simulink model "ISA_simulation"  (R2018b)
settings: Solver=FixedStepDiscrete  StartTime=0.0  StopTime=10  FixedStep=0.01  RelTol=1e-3
PreLoadFcn:
  | librarySetup
  | eval([bdroot,'_startup']) %Calling [modelName]_startup.m
InitFcn:
  | ISA_simulation_startup
values from neighbouring files (symbols this model uses):
  Error_detection = -1    [ISA_simulation_startup.m]
  ID727_Byte0 = 50    [ISA_simulation_startup.m]
  ID727_Byte1 = 0    [ISA_simulation_startup.m]
  ID727_Byte2 = 0    [ISA_simulation_startup.m]
  ID727_Byte3 = 0    [ISA_simulation_startup.m]
  ID727_Byte4 = 0    [ISA_simulation_startup.m]
  ID727_Byte5 = 0    [ISA_simulation_startup.m]
  ID727_Byte6 = 0    [ISA_simulation_startup.m]
  ID727_Byte7 = 0    [ISA_simulation_startup.m]
  ID7E8_Byte0 = 3    [ISA_simulation_startup.m]
  ID7E8_Byte1 = 65    [ISA_simulation_startup.m]
  ID7E8_Byte2 = 13    [ISA_simulation_startup.m]
  ID7E8_Byte3 = 2    [ISA_simulation_startup.m]
  ID7E8_Byte4 = 0    [ISA_simulation_startup.m]
  ID7E8_Byte5 = 0    [ISA_simulation_startup.m]
  ID7E8_Byte6 = 0    [ISA_simulation_startup.m]
  ID7E8_Byte7 = 0    [ISA_simulation_startup.m]
  PWM_motor = 0.6    [ISA_simulation_startup.m]    (also in ISA_startup.m = 0.55)
undefined symbols (not defined in the file or in its folder): DiscIntNeverNeededParam
libraries: simulink x14, HANcoder_STM32_Target x5, HANcoder_STM32_Target2009b x2, simulink_extras x1
CloseFcn:
  | rtwprivate ssgencode ModelCloseRequest mytest
settings Model: Creator=Saliou  LastModifiedBy=Saliou
settings SolverCC: PositivePriorityOrder=on
settings DataIOCC: LimitDataPoints=on  SaveFormat=Array  SaveOutput=off  SaveTime=off
settings OptimizationCC: BlockReduction=off  DefaultParameterBehavior=Inlined  DefaultUnderspecifiedDataType=single  InlineInvariantSignals=on  ExpressionDepthLimit=2147483647  StateBitsets=on  DataBitsets=on  ZeroExternalMemoryAtStartup=off  ZeroInternalMemoryAtStartup=off  InitFltsAndDblsToZero=on  NoFixptDivByZeroProtection=on  EfficientFloat2IntCast=on  LifeSpan=inf
settings DebuggingCC: SaveWithDisabledLinksMsg=none  SaveWithParameterizedLinksMsg=none  CheckSSInitialOutputMsg=off  UnderspecifiedInitializationDetection=Classic  MergeDetectMultiDrivingBlocksExec=none  SignalResolutionControl=TryResolveAll  SolverPrmCheckMsg=warning  InheritedTsInSrcMsg=none  MultiTaskDSMMsg=warning  MultiTaskCondExecSysMsg=none  ParameterPrecisionLossMsg=none  FcnCallInpInsideContextMsg=warning  StateNameClashWarn=warning  SFUnexpectedBacktrackingDiag=warning  SFNoUnconditionalDefaultTransitionDiag=warning  SFExecutionAtInitializationDiag=none
settings HardwareCC: ProdBitPerPointer=32  ProdBitPerSizeT=32  ProdBitPerPtrDiffT=32  ProdLargestAtomicInteger=Long  ProdLargestAtomicFloat=Double  ProdWordSize=32  ProdHWDeviceType=ARM Compatible->ARM Cortex  TargetEndianess=LittleEndian  TargetHWDeviceType=Infineon->TriCore
settings ModelReferenceCC: PropagateSignalLabelsOutOfModel=off
settings SFSimCC: SimUseLocalCustomCode=off  MATLABDynamicMemAlloc=off
settings RTWCC: SystemTargetFile=ert.tlc  MakeCommand=make_rtw SHELL= HANcoder_PORTABLE=1 HANcoder_BOOTLOADER=1  TemplateMakefile=Olimexino_STM32_gcc.tmf  Description=Real-Time Workshop Embedded Coder (no auto configuration)  RTWUseLocalCustomCode=off
settings CodeAppCC: ForceParamTrailComments=on  IgnoreCustomStorageClasses=off  SimulinkDataObjDesc=on  CustomSymbolStrGlobalVar=rt$N$M  CustomSymbolStrType=$N$M  CustomSymbolStrFcn=$N$M$F  CustomSymbolStrMacro=$N$M  InsertBlockDesc=on  StateflowObjectComments=on  InternalIdentifier=Classic
settings ERTTargetCC: TargetFcnLib=ansi_tfl_tmw.mat  MultiwordLength=2048  IncludeMdlTerminateFcn=off  SuppressErrorStatus=on  SupportNonFinite=off  GenerateASAP2=on  InlinedParameterPlacement=NonHierarchical  ERTCustomFileTemplate=example_file_process.tlc  ConvertIfToSwitch=off  SuppressUnreachableDefaultCases=off
settings ConfigComp: CovMetricSettings=dw  CovHtmlReporting=on  CovSaveCumulativeToWorkspaceVar=on  CovSaveSingleToWorkspaceVar=on  CovExternalEMLEnable=off  CovSFcnEnable=off  DVMaxProcessTime=600  DVDisplayUnsatisfiableObjectives=on  DVAutomaticStubbing=off  DVModelCoverageObjectives=MCDC  DVMaxTestCaseSteps=500  DVTestSuiteOptimization=CombinedObjectives  DVDetectActiveLogic=on  DVSaveHarnessModel=on

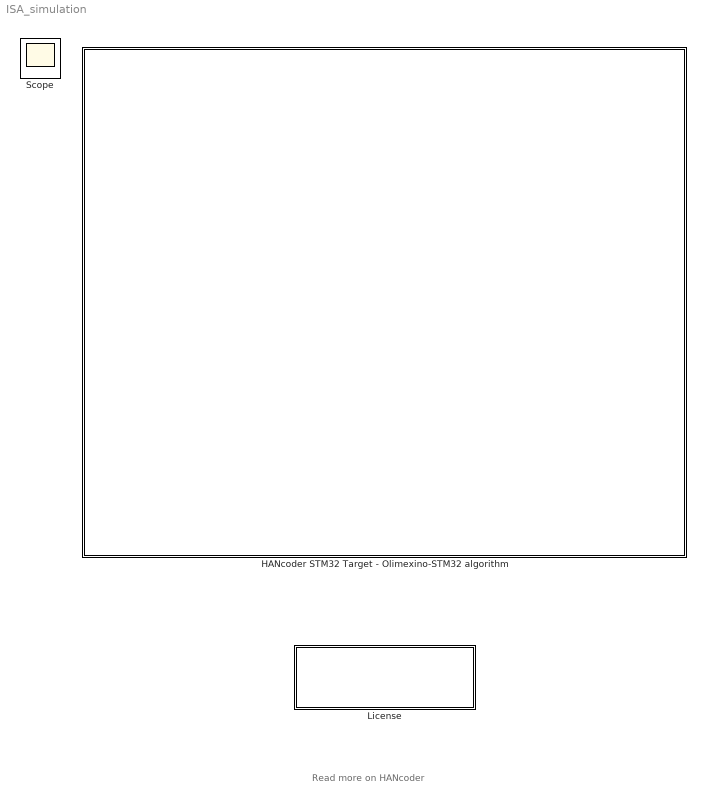
== system ISA_simulation ==
  note: Read more on HANcoder
  HANcoder STM32 Target - Olimexino-STM32 algorithm : Subsystem  mask(TopLevelSubsystem){}
      settings: CopyFcn=HANcoderChecks('Copy');  NameChangeFcn=HANcoderChecks('NameChangeOlimexino');  MoveFcn=HANcoderChecks('MoveOlimexino');
      mask Display: image(imread('Olimexino_STM32_HAN.jpg'))
  License : Subsystem  mask(License){}
      settings: NameChangeFcn=HANcoderChecks('NameChangeLicenseBlock');  OpenFcn=winopen('License.pdf')  MoveFcn=HANcoderChecks('MoveLicenseBlock');
      mask Display: disp(['End-User License Agreement\n','please read before use']);
  Scope : Scope

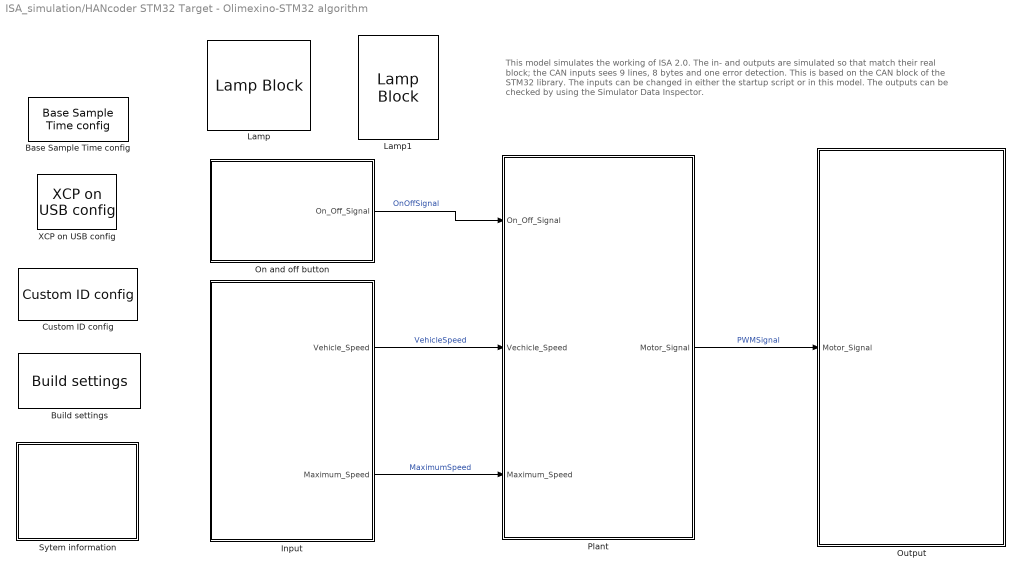
== system ISA_simulation/HANcoder STM32 Target - Olimexino-STM32 algorithm ==
  note: This model simulates the working of ISA 2.0. The in- and outputs are simulated so that match their real
      | block; the CAN inputs sees 9 lines, 8 bytes and one error detection. This is based on the CAN block of the
      | STM32 library. The inputs can be changed in either the startup script or in this model. The outputs can be
      | checked by using the Simulator Data Inspector.
  Base Sample Time config : HANcoder_STM32_Target/Olimexino STM32/System Config/Base Sample Time config  Tag=HANcoder_TARGET_STM32_Olimexino  Description=HANcoder Target STM32-Olimexino blockset version 1.0  baseSampleTime=10  extraStack=0
      settings: SourceProductName=HANcoder STM32 Target
  Build settings : HANcoder_STM32_Target/Olimexino STM32/System Config/Build settings  Tag=HANcoder_TARGET_STM32_Olimexino  AutoASAP2add=on  AutoFlash=USB
      settings: SourceProductName=HANcoder STM32 Target
  Custom ID config : HANcoder_STM32_Target2009b/Olimexino STM32/System Config/Custom ID config  Tag=HANcoder_TARGET_STM32_Olimexino  softID=softwareID  softNUM=1
  Input : Subsystem
  Lamp : LampBlock  WebBlockId=3805
  Lamp1 : LampBlock  WebBlockId=3832
  On and off button : Subsystem
  Output : Subsystem
  Plant : Subsystem
  Sytem information : Subsystem
  XCP on USB config : HANcoder_STM32_Target2009b/Olimexino STM32/System Config/XCP on USB config  Tag=HANcoder_TARGET_STM32_Olimexino
  wires:
  Input/2(Maximum_Speed) -> Plant/3(Maximum_Speed)  "MaximumSpeed"
  Input/1(Vehicle_Speed) -> Plant/2(Vechicle_Speed)  "VehicleSpeed"
  Plant/1(Motor_Signal) -> Output/1(Motor_Signal)  "PWMSignal"
  On and off button/1(On_Off_Signal) -> Plant/1(On_Off_Signal)  "OnOffSignal"

== system ISA_simulation/License ==

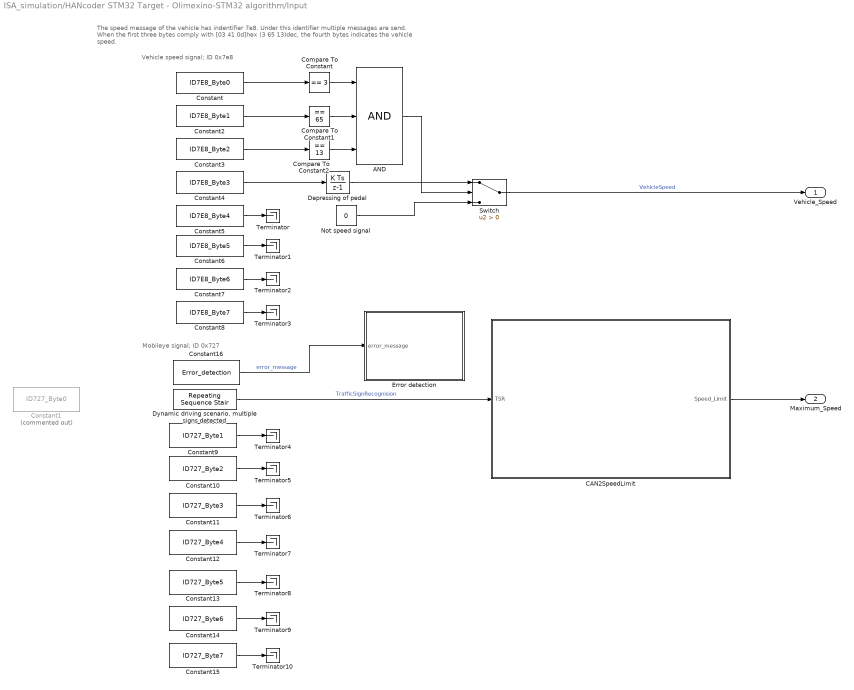
== system ISA_simulation/HANcoder STM32 Target - Olimexino-STM32 algorithm/Input ==
  note: Mobileye signal; ID 0x727
  note: Vehicle speed signal; ID 0x7e8
  note: The speed message of the vehicle has indentifier 7e8. Under this identifier multiple messages are send. When the first three bytes comply with [03 41 0d]hex (3 65 13)dec, the fourth bytes indicates the vehicle speed.
  AND : Logic  Inputs=3  AllPortsSameDT=off  OutDataTypeStr=boolean
  CAN2SpeedLimit : Subsystem
  Compare To Constant : simulink/Logic and Bit Operations/Compare To Constant  relop===  const=3  OutDataTypeStr=boolean
  Compare To Constant1 : simulink/Logic and Bit Operations/Compare To Constant  relop===  const=65  OutDataTypeStr=boolean
  Compare To Constant2 : simulink/Logic and Bit Operations/Compare To Constant  relop===  const=13  OutDataTypeStr=boolean
  Constant : Constant  Value=ID7E8_Byte0
  Constant1 : Constant  Commented=on  Value=ID727_Byte0  OutDataTypeStr=single
  Constant10 : Constant  Value=ID727_Byte2  OutDataTypeStr=single
  Constant11 : Constant  Value=ID727_Byte3  OutDataTypeStr=single
  Constant12 : Constant  Value=ID727_Byte4  OutDataTypeStr=single
  Constant13 : Constant  Value=ID727_Byte5  OutDataTypeStr=single
  Constant14 : Constant  Value=ID727_Byte6  OutDataTypeStr=single
  Constant15 : Constant  Value=ID727_Byte7  OutDataTypeStr=single
  Constant16 : Constant  Value=Error_detection  OutDataTypeStr=single
  Constant2 : Constant  Value=ID7E8_Byte1
  Constant3 : Constant  Value=ID7E8_Byte2
  Constant4 : Constant  Value=ID7E8_Byte3  OutDataTypeStr=single
  Constant5 : Constant  Value=ID7E8_Byte4  OutDataTypeStr=single
  Constant6 : Constant  Value=ID7E8_Byte5  OutDataTypeStr=single
  Constant7 : Constant  Value=ID7E8_Byte6  OutDataTypeStr=single
  Constant8 : Constant  Value=ID7E8_Byte7  OutDataTypeStr=single
  Constant9 : Constant  Value=ID727_Byte1  OutDataTypeStr=single
  Depressing of pedal : DiscreteIntegrator  gainval=13  SampleTime=-1  ICPrevOutput=DiscIntNeverNeededParam  ICPrevScaledInput=DiscIntNeverNeededParam
  "Dynamic driving scenario, multiple signs detected" : simulink/Sources/Repeating Sequence Stair  OutValues=[2 7 4 12 9].'  tsamp=1  OutMin=[]  OutMax=[]  OutDataTypeStr=double  OutputDataTypeScalingMode=double  OutDataType=fixdt(0,8)  ConRadixGroup=Best Precision: Vector-wise  OutScaling=2^-12
  Error detection : Subsystem
  Not speed signal : Constant  Value=0
  Switch : Switch  Criteria=u2 > Threshold
  Terminator{,1..10} (11 alike) : Terminator
  Vehicle_Speed : Outport
  Maximum_Speed : Outport  Port=2
  wires:
  Switch/1 -> Vehicle_Speed/1  "VehicleSpeed"
  Constant/1 -> Compare To Constant/1
  Constant2/1 -> Compare To Constant1/1
  Constant3/1 -> Compare To Constant2/1
  Compare To Constant2/1 -> AND/3
  Compare To Constant1/1 -> AND/2
  Compare To Constant/1 -> AND/1
  AND/1 -> Switch/2
  Not speed signal/1 -> Switch/3
  Constant5/1 -> Terminator/1
  Constant6/1 -> Terminator1/1
  Constant7/1 -> Terminator2/1
  Constant8/1 -> Terminator3/1
  Constant9/1 -> Terminator4/1
  Constant10/1 -> Terminator5/1
  Constant11/1 -> Terminator6/1
  Constant12/1 -> Terminator7/1
  Constant13/1 -> Terminator8/1
  Constant14/1 -> Terminator9/1
  Constant15/1 -> Terminator10/1
  Constant4/1 -> Depressing of pedal/1
  Depressing of pedal/1 -> Switch/1
  "Dynamic driving scenario, multiple signs detected"/1 -> CAN2SpeedLimit/1(TSR)  "TrafficSignRecognision"
  CAN2SpeedLimit/1(Speed_Limit) -> Maximum_Speed/1
  Constant16/1 -> Error detection/1(error_message)  "error_message"

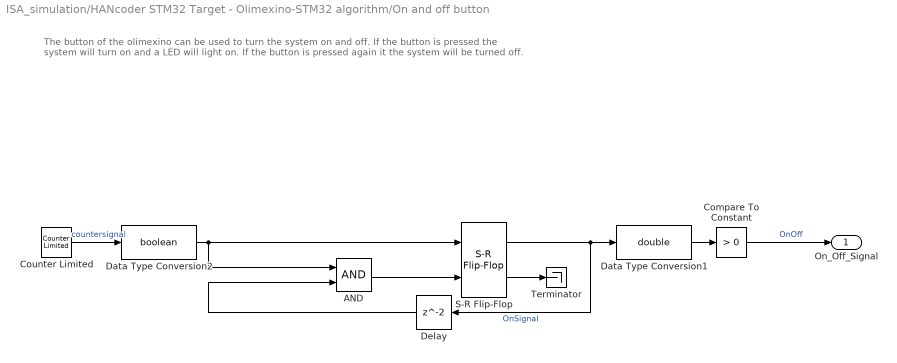
== system ISA_simulation/HANcoder STM32 Target - Olimexino-STM32 algorithm/On and off button ==
  note: The button of the olimexino can be used to turn the system on and off. If the button is pressed the system will turn on and a LED will light on. If the button is pressed again it the system will be turned off.
  AND : Logic  AllPortsSameDT=off  OutDataTypeStr=boolean
  Compare To Constant : simulink/Logic and Bit Operations/Compare To Constant  relop=>  const=0  OutDataTypeStr=boolean
  Counter Limited : simulink/Sources/Counter Limited  uplimit=1  tsamp=1
  Data Type Conversion1 : DataTypeConversion  OutDataTypeStr=double
  Data Type Conversion2 : DataTypeConversion  OutDataTypeStr=boolean
  Delay : Delay
  S-R Flip-Flop : simulink_extras/Flip Flops/S-R Flip-Flop  initial_condition=0
  Terminator : Terminator
  On_Off_Signal : Outport
  wires:
  AND/1 -> S-R Flip-Flop/2
  Data Type Conversion2/1 -> AND/1, S-R Flip-Flop/1
  Counter Limited/1 -> Data Type Conversion2/1  "countersignal"
  S-R Flip-Flop/1 -> Delay/1, Data Type Conversion1/1  "OnSignal"
  Data Type Conversion1/1 -> Compare To Constant/1
  Compare To Constant/1 -> On_Off_Signal/1  "OnOff"
  S-R Flip-Flop/2 -> Terminator/1
  Delay/1 -> AND/2

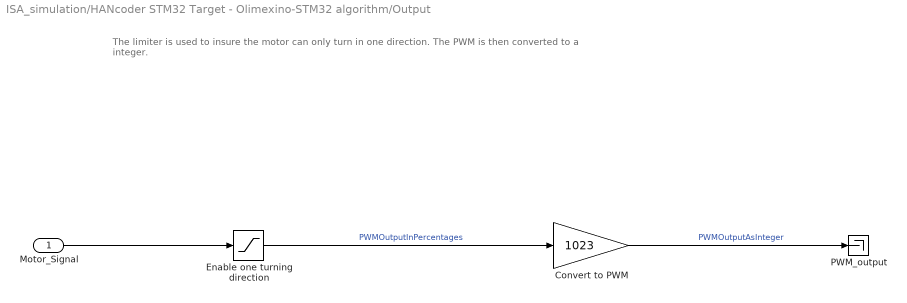
== system ISA_simulation/HANcoder STM32 Target - Olimexino-STM32 algorithm/Output ==
  note: The limiter is used to insure the motor can only turn in one direction. The PWM is then converted to a integer.
  Motor_Signal : Inport
  Convert to PWM : Gain  Gain=1023
  Enable one turning direction : Saturate  UpperLimit=0.6  LowerLimit=0
  PWM_output : Terminator
  wires:
  Motor_Signal/1 -> Enable one turning direction/1
  Enable one turning direction/1 -> Convert to PWM/1  "PWMOutputInPercentages"
  Convert to PWM/1 -> PWM_output/1  "PWMOutputAsInteger"

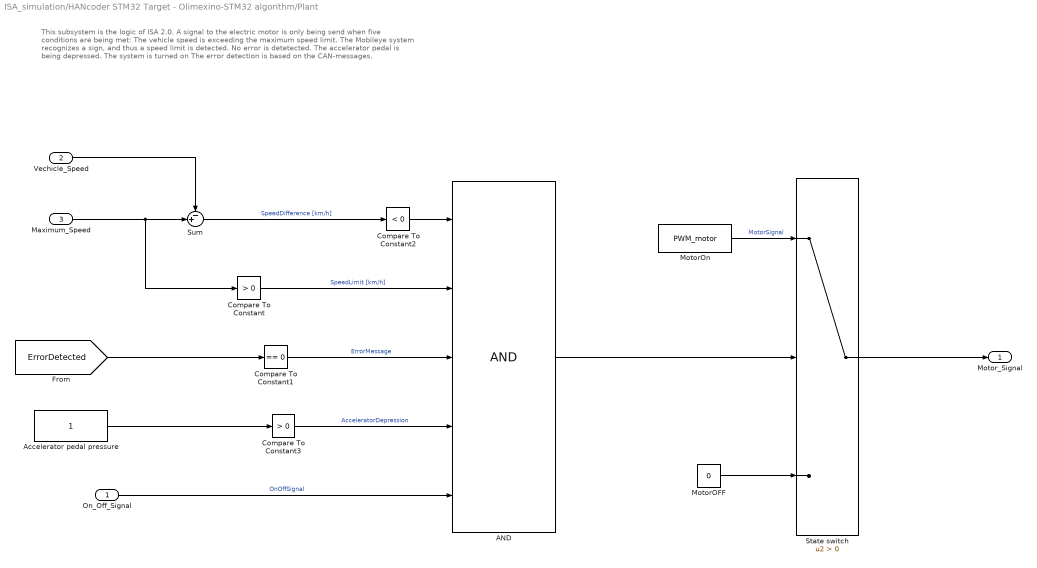
== system ISA_simulation/HANcoder STM32 Target - Olimexino-STM32 algorithm/Plant ==
  note: This subsystem is the logic of ISA 2.0. A signal to the electric motor is only being send when five conditions are being met:
      | The vehicle speed is exceeding the maximum speed limit.
      | The Mobileye system recognizes a sign, and thus a speed limit is detected.
      | No error is detetected.
      | The accelerator pedal is being depressed.
      | The system is turned on
      | The error detection is based on the CAN-messages.
  On_Off_Signal : Inport
  Vechicle_Speed : Inport  Port=2
  Maximum_Speed : Inport  Port=3
  AND : Logic  Inputs=5  AllPortsSameDT=off  OutDataTypeStr=boolean
  Accelerator pedal pressure : Constant
  Compare To Constant : simulink/Logic and Bit Operations/Compare To Constant  relop=>  const=0  OutDataTypeStr=boolean
  Compare To Constant1 : simulink/Logic and Bit Operations/Compare To Constant  relop===  const=0  OutDataTypeStr=boolean
  Compare To Constant2 : simulink/Logic and Bit Operations/Compare To Constant  relop=<  const=0  OutDataTypeStr=boolean
  Compare To Constant3 : simulink/Logic and Bit Operations/Compare To Constant  relop=>  const=0  OutDataTypeStr=boolean
  MotorOFF : Constant  Value=0
  MotorOn : Constant  Value=PWM_motor
  State switch : Switch  Criteria=u2 > Threshold
  Sum : Sum  Inputs=-+|
  Motor_Signal : Outport
  wires:
  State switch/1 -> Motor_Signal/1
  MotorOn/1 -> State switch/1  "MotorSignal"
  Sum/1 -> Compare To Constant2/1  "SpeedDifference [km/h]"
  Maximum_Speed/1 -> Compare To Constant/1, Sum/2
  Vechicle_Speed/1 -> Sum/1
  MotorOFF/1 -> State switch/3
  Compare To Constant/1 -> AND/2  "SpeedLimit [km/h]"
  AND/1 -> State switch/2
  [ErrorDetected] -> Compare To Constant1/1
  Compare To Constant1/1 -> AND/3  "ErrorMessage"
  Compare To Constant2/1 -> AND/1
  Compare To Constant3/1 -> AND/4  "AcceleratorDepression"
  Accelerator pedal pressure/1 -> Compare To Constant3/1
  On_Off_Signal/1 -> AND/5  "OnOffSignal"

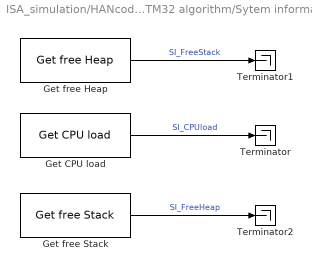
== system ISA_simulation/HANcoder STM32 Target - Olimexino-STM32 algorithm/Sytem information ==
  Get CPU load : HANcoder_STM32_Target/Olimexino STM32/System Management/Get CPU load  Tag=HANcoder_TARGET_STM32_Olimexino  mode=Current CPU load  tsamp=-1
      settings: SourceProductName=HANcoder STM32 Target
  Get free Heap : HANcoder_STM32_Target/Olimexino STM32/System Management/Get free Heap  Tag=HANcoder_TARGET_STM32_Olimexino  tsamp=-1
      settings: SourceProductName=HANcoder STM32 Target
  Get free Stack : HANcoder_STM32_Target/Olimexino STM32/System Management/Get free Stack  Tag=HANcoder_TARGET_STM32_Olimexino  taskIdx=Application Control Task  tsamp=-1
      settings: SourceProductName=HANcoder STM32 Target
  Terminator : Terminator
  Terminator1 : Terminator
  Terminator2 : Terminator
  wires:
  Get CPU load/1 -> Terminator/1  "SI_CPUload"
  Get free Heap/1 -> Terminator1/1  "SI_FreeStack"
  Get free Stack/1 -> Terminator2/1  "SI_FreeHeap"

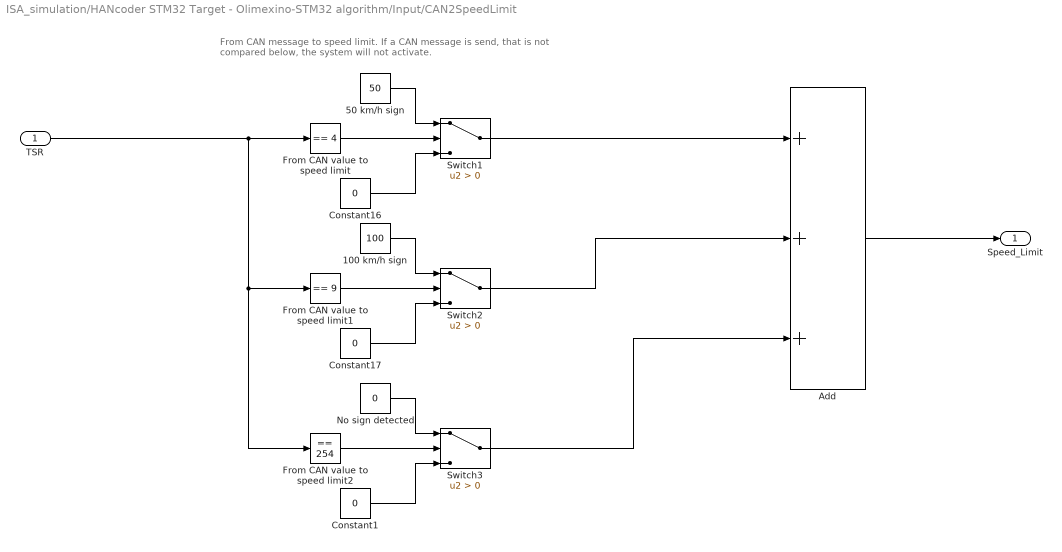
== system ISA_simulation/HANcoder STM32 Target - Olimexino-STM32 algorithm/Input/CAN2SpeedLimit ==
  note: From CAN message to speed limit. If a CAN message is send,
      | that is not compared below, the system will not activate.
  TSR : Inport
  100 km/h sign : Constant  Value=100
  50 km/h sign : Constant  Value=50
  Add : Sum  Inputs=+++
  Constant1 : Constant  Value=0
  Constant16 : Constant  Value=0
  Constant17 : Constant  Value=0
  From CAN value to speed limit : simulink/Logic and Bit Operations/Compare To Constant  relop===  const=4  OutDataTypeStr=boolean
  From CAN value to speed limit1 : simulink/Logic and Bit Operations/Compare To Constant  relop===  const=9  OutDataTypeStr=boolean
  From CAN value to speed limit2 : simulink/Logic and Bit Operations/Compare To Constant  relop===  const=254  OutDataTypeStr=boolean
  No sign detected : Constant  Value=0
  Switch1 : Switch  Criteria=u2 > Threshold
  Switch2 : Switch  Criteria=u2 > Threshold
  Switch3 : Switch  Criteria=u2 > Threshold
  Speed_Limit : Outport
  wires:
  Constant17/1 -> Switch2/3
  100 km/h sign/1 -> Switch2/1
  Switch2/1 -> Add/2
  Constant16/1 -> Switch1/3
  From CAN value to speed limit1/1 -> Switch2/2
  Switch1/1 -> Add/1
  From CAN value to speed limit/1 -> Switch1/2
  50 km/h sign/1 -> Switch1/1
  Add/1 -> Speed_Limit/1
  Constant1/1 -> Switch3/3
  No sign detected/1 -> Switch3/1
  From CAN value to speed limit2/1 -> Switch3/2
  Switch3/1 -> Add/3
  TSR/1 -> From CAN value to speed limit2/1, From CAN value to speed limit1/1, From CAN value to speed limit/1

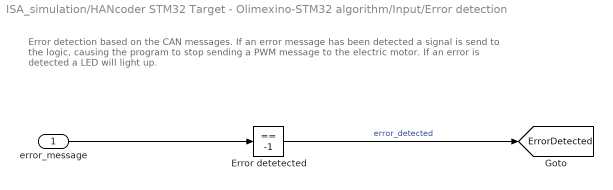
== system ISA_simulation/HANcoder STM32 Target - Olimexino-STM32 algorithm/Input/Error detection ==
  note: Error detection based on the CAN messages. If an error message has been detected a signal is send to the logic, causing the program
      | to stop sending a PWM message to the electric motor. If an error is detected a LED will light up.
  error_message : Inport
  Error detetected : simulink/Logic and Bit Operations/Compare To Constant  relop===  const=-1  OutDataTypeStr=boolean
  tag scope: ErrorDetected=global
  wires:
  error_message/1 -> Error detetected/1
  Error detetected/1 -> [ErrorDetected]  "error_detected"
